simulink model "Liveness"  (R2021b)
settings: Solver=FixedStepDiscrete  StartTime=0.0  StopTime=10.0  FixedStep=0.1  RelTol=1e-3  EnableMultiTasking=on
undefined symbols (not defined in the file or in its folder): sldvsubsys
libraries: sldvlib x2, hdlsllib x2, simulink x1
settings Model: DVExtractedSubsystem=Liveness  Creator=Alessandro  LastModifiedBy=Alessandro
settings SolverCC: AlgebraicLoopSolver=TrustRegion  AutoInsertRateTranBlk=on
settings DataIOCC: LimitDataPoints=on
settings OptimizationCC: LifeSpan=inf
settings DebuggingCC: FrameProcessingCompatibilityMsg=none  AllowSymbolicDim=off  SFUnexpectedBacktrackingDiag=warning  SFNoUnconditionalDefaultTransitionDiag=warning  SFExecutionAtInitializationDiag=none  ArithmeticOperatorsInVariantConditions=warning
settings SFSimCC: SimUseLocalCustomCode=off  CustomCodeUndefinedFunction=UseInterfaceOnly
settings RTWCC: RTWUseLocalCustomCode=off
settings CodeAppCC: StateflowObjectComments=on
settings GRTTargetCC: TargetLangStandard=C89/C90 (ANSI)
settings ConfigComp: CovMetricSettings=dw  CovSaveCumulativeToWorkspaceVar=on  CovSaveSingleToWorkspaceVar=on  CovExternalEMLEnable=off  CovSFcnEnable=off  DVMode=PropertyProving  DVTestSuiteOptimization=Auto  DVDetectOutOfBounds=on  DVModelReferenceHarness=on

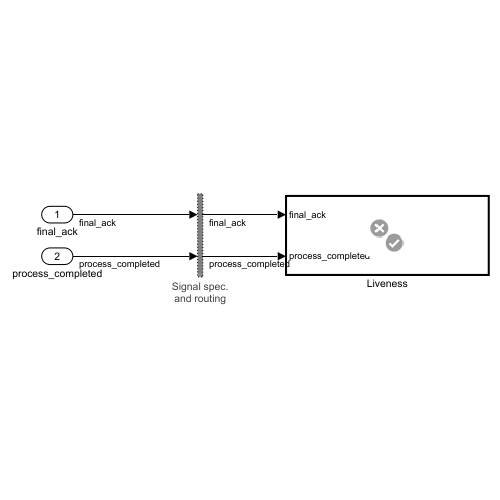
[thumbnail: Simulink's stored preview of the top-level diagram]
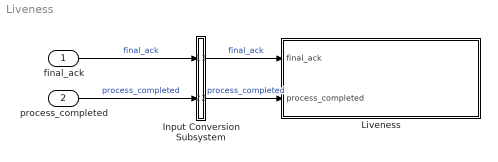
== system Liveness ==
  final_ack : Inport  OutDataTypeStr=double  PortDimensions=[1]  SampleTime=0.1  Interpolate=off
  process_completed : Inport  Port=2  OutDataTypeStr=double  PortDimensions=[1]  SampleTime=0.1  Interpolate=off
  Input Conversion Subsystem : Subsystem  Tag=__SLT_ICS__  Description=|
      | Signal spec.
      | and routing
      settings: AttributesFormatString=%<Description>
  Liveness : Subsystem  Tag=VerificationSubsystem  DisableCoverage=on  LoadFcn=sldvsubsys('check')  TreatAsAtomicUnit=on  SimViewingDevice=on  mask(VerificationSubsystem){}
      mask init:
      | sldvsubsys('maskInit');
      settings: CopyFcn=sldvsubsys('copy');  OpenFcn=open_system(gcb,'force');
      settings: PreSaveFcn=|
      | set_param(gcb,'SimViewingDevice','on');
      | sldvsubsys('check');
      mask Help: helpview(fullfile(docroot,'toolbox','sldv','sldv.map'),'verificationsubsystem')
      mask Display: image(imread('sldvicon_versubsys.png','BackGroundColor',[1 1 1]),'center');
  wires:
  final_ack/1 -> Input Conversion Subsystem/1(Inport_1)  "final_ack"
  process_completed/1 -> Input Conversion Subsystem/2(Inport_2)  "process_completed"
  Input Conversion Subsystem/1(Outport_1) -> Liveness/1(final_ack)  "final_ack"
  Input Conversion Subsystem/2(Outport_2) -> Liveness/2(process_completed)  "process_completed"

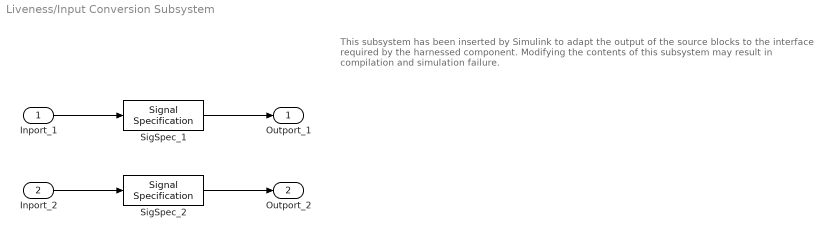
== system Liveness/Input Conversion Subsystem ==
  note: This subsystem has been inserted by Simulink to adapt the output of the source blocks to the interface required by the harnessed component.
      |  Modifying the contents of this subsystem may result in compilation and simulation failure.
  Inport_1 : Inport
  Inport_2 : Inport  Port=2
  SigSpec_1 : SignalSpecification  OutDataTypeStr=double  Dimensions=[1]  SampleTime=0.1
  SigSpec_2 : SignalSpecification  OutDataTypeStr=double  Dimensions=[1]  SampleTime=0.1
  Outport_1 : Outport
  Outport_2 : Outport  Port=2
  wires:
  SigSpec_1/1 -> Outport_1/1
  Inport_1/1 -> SigSpec_1/1
  SigSpec_2/1 -> Outport_2/1
  Inport_2/1 -> SigSpec_2/1

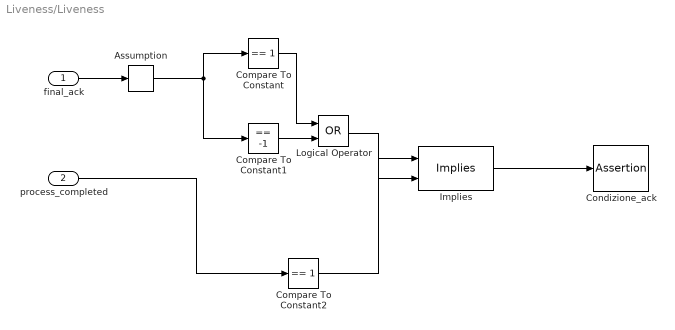
== system Liveness/Liveness ==
  final_ack : Inport  OutDataTypeStr=double
  process_completed : Inport  Port=2  OutDataTypeStr=double
  Assumption : sldvlib/Objectives and Constraints/Assumption  enabled=off  customAVTBlockType=Assumption  intervals={-1,1}  initial=off  dispValues=on  outEnabled=on
      settings: AttributesFormatString=%<intervals>  SourceProductBaseCode=SL
  Compare To Constant : hdlsllib/Logic and Bit Operations/Compare To Constant  relop===  const=1  OutDataTypeStr=boolean
      settings: SourceProductBaseCode=SL
  Compare To Constant1 : hdlsllib/Logic and Bit Operations/Compare To Constant  relop===  const=-1  OutDataTypeStr=boolean
      settings: SourceProductBaseCode=SL
  Compare To Constant2 : simulink/Logic and Bit Operations/Compare To Constant  relop===  const=1  OutDataTypeStr=boolean
  Condizione_ack : Assertion  StopWhenAssertionFail=off
  Implies : sldvlib/Verification Utilities/Implies
      settings: SourceProductBaseCode=SL
  Logical Operator : Logic  Operator=OR  AllPortsSameDT=off  OutDataTypeStr=boolean
  wires:
  Logical Operator/1 -> Implies/2
  Compare To Constant1/1 -> Logical Operator/2
  Compare To Constant/1 -> Logical Operator/1
  Assumption/1 -> Compare To Constant/1, Compare To Constant1/1
  Implies/1 -> Condizione_ack/1
  Compare To Constant2/1 -> Implies/1
  process_completed/1 -> Compare To Constant2/1
  final_ack/1 -> Assumption/1
